simulink model "sourceLocalization_ol"  (R2020a)
settings: Solver=VariableStepAuto  StartTime=0.0  StopTime=inf  RelTol=1e-3
model workspace (MAT data in the model file):
  VADThreshold = 0.5
  c0 = 348
  elementSpace = 0.275
  frameLength = 9600
  fs = 96000
undefined symbols (not defined in the file or in its folder): phased
libraries: dspnetwork x6, audiomeasurements x4, dspstat3 x2, audiosources x1, dspsnks4 x1, dspsrcs4 x1, dspvision x1, dspsigops x1, simulink x1
settings Model: OrderedModelArguments=off  Creator=GH  LastModifiedBy=GH
settings DebuggingCC: UnderSpecifiedDimensionMsg=warning

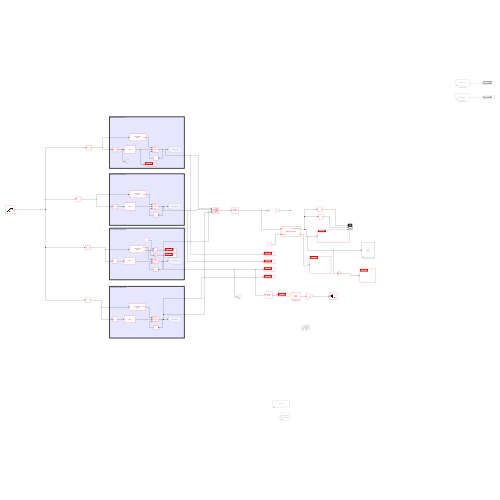
[thumbnail: Simulink's stored preview of the top-level diagram]
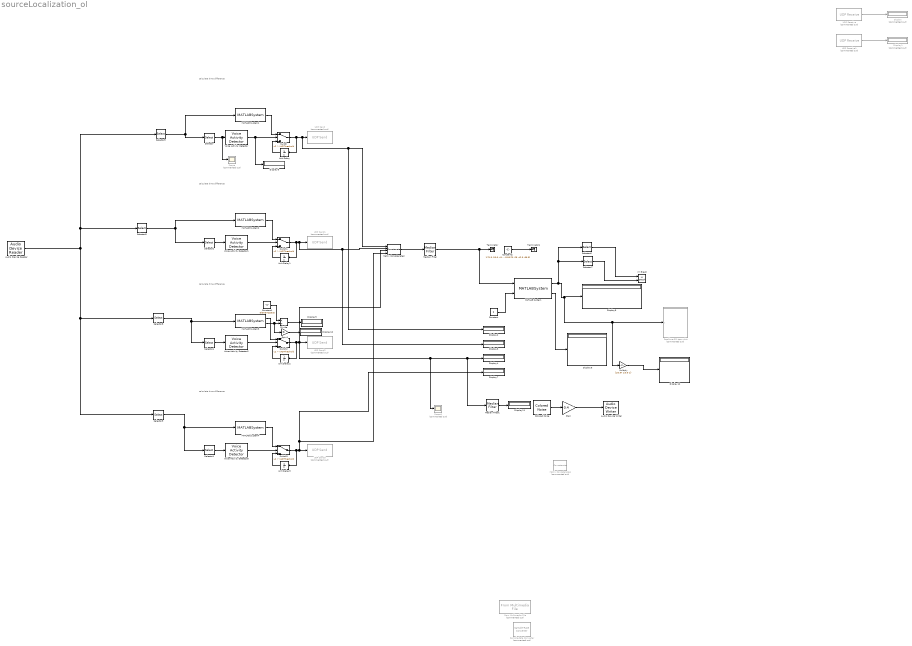
== system sourceLocalization_ol ==
  note: calculate time difference
  note: calculate time difference
  note: calculate time difference
  note: calculate time difference
  Audio Device Reader : audiosources/Audio Device Reader  Driver=ASIO  Device=Default  SampleRate=fs  NumChannels=8  SamplesPerFrame=frameLength  BitDepth=16-bit integer  NumBuffers=10  DefaultInputChannelMapping=on  InputChannelMapping=1:2  OutputNumOverrunSamples=off  OutputDataType=double  DriverIdx=3  DeviceWarnFlag=''
      settings: SourceProductBaseCode=AU
  Audio Device Writer : dspsnks4/Audio Device Writer  Driver=ASIO  Device=Default  InheritSampleRate=on  SampleRate=44100  BitDepth=16-bit integer  BufferSize=4096  NumBuffers=10  DefaultOutputChannelMapping=on  OutputChannelMapping=1:2  OutputNumUnderrunSamples=off  DriverIdx=3  DeviceWarnFlag=''
  Colored Noise : dspsrcs4/Colored Noise  Color=pink  InverseFrequencyPower=1  BoundedOutput=on  NumChannels=1  OutputDataType=double  SamplesPerFrame=frameLength  SampleTime=1/fs  RandomStream=mt19937ar with seed  Seed=67  SimulateUsing=Interpreted execution
      settings: SourceProductBaseCode=DS
  Constant : Constant
  Constant1 : Constant  Value=elementSpace
  Constant2 : Constant  Value=1*[1.5 -26.6 -41.4 -57.9]+0*[0 -28 -42.9 -56.9]  VectorParams1D=off
  Display : Display  Commented=on
  Display1 : Display  Commented=on
  Display{2..12} (11 alike) : Display
  Divide : Product  Inputs=*/
  From Multimedia File : dspvision/From Multimedia File  Commented=on  inputFilename=/Users/developer/Downloads/tan.wav  readRange=[1 Inf]  loop=on  numPlays=inf  outputStreams=Audio only  videoDataType=single  audioDataType=double  inheritSampleTime=on  userDefinedSampleTime=1/30  noAudioOutput=off  isIntensityVideo=off  fourcc=RGB  colorVideoFormat=Separate color signals  outputEOF=off  dataOrg=Column-major  audioFrameSize=frameLength  computeAudioFrameSize=off  outSamplingMode=Sample based
  Gain : Gain  Gain=0.4
  Gain1 : Gain  Gain=fs
  MATLAB System : MATLABSystem  System=getSourcePosition  arrayPos=arrayPos  arrayAxis=arrayAxis  maxStepLength=0.1  sourcePos0=[2;5;2]  SimulateUsing=Interpreted execution
      mask Type: getSourcePosition
      mask Display:
      | disp('getSourcePosition');
      | port_label('input',1,'aoa');
      | port_label('input',2,'calFlag');
      | port_label('output',1,'sourcePosition');
      | port_label('output',2,'dr');
  MATLAB System1 : MATLABSystem  System=GCCEstimator  PropagationSpeed=c0  SampleRateFromInputCheckbox=on  SampleRate=1e6  SensorPairSource=Auto  SensorPair=[ 2; 1 ]  CorrelationOutputPort=off  DelayOutputPort=off  SimulateUsing=Interpreted execution  SensorArray=phased.ULA('Element',phased.OmnidirectionalMicrophoneElement(),'ElementSpacing',elementSpace)
      mask Type: GCCEstimator
      mask Display:
      | disp(['GCC-PHAT' char(10) 'DOA']);
      | port_label('output',1,'Ang');
  MATLAB System2 : MATLABSystem  System=GCCEstimator  PropagationSpeed=c0  SampleRateFromInputCheckbox=on  SampleRate=1e6  SensorPairSource=Auto  SensorPair=[ 2; 1 ]  CorrelationOutputPort=off  DelayOutputPort=off  SimulateUsing=Interpreted execution  SensorArray=phased.ULA('Element',phased.OmnidirectionalMicrophoneElement(),'ElementSpacing',elementSpace)
      mask Type: GCCEstimator
      mask Display:
      | disp(['GCC-PHAT' char(10) 'DOA']);
      | port_label('output',1,'Ang');
  MATLAB System3 : MATLABSystem  System=GCCEstimator  PropagationSpeed=c0  SampleRateFromInputCheckbox=on  SampleRate=1e6  SensorPairSource=Auto  SensorPair=[ 2; 1 ]  CorrelationOutputPort=off  DelayOutputPort=on  SimulateUsing=Interpreted execution  SensorArray=phased.ULA('Element',phased.OmnidirectionalMicrophoneElement(),'ElementSpacing',elementSpace)
      mask Type: GCCEstimator
      mask Display:
      | disp(['GCC-PHAT' char(10) 'DOA']);
      | port_label('output',1,'Ang');
      | port_label('output',2,'Tau');
  MATLAB System4 : MATLABSystem  System=GCCEstimator  PropagationSpeed=c0  SampleRateFromInputCheckbox=on  SampleRate=1e6  SensorPairSource=Auto  SensorPair=[ 2; 1 ]  CorrelationOutputPort=off  DelayOutputPort=off  SimulateUsing=Interpreted execution  SensorArray=phased.ULA('Element',phased.OmnidirectionalMicrophoneElement(),'ElementSpacing',elementSpace)
      mask Type: GCCEstimator
      mask Display:
      | disp(['GCC-PHAT' char(10) 'DOA']);
      | port_label('output',1,'Ang');
  Matrix Concatenate1 : Concatenate  Commented=on  Mode=Multidimensional array  ConcatenateDimension=2
  Matrix Concatenate2 : Concatenate  NumInputs=4  Mode=Multidimensional array  ConcatenateDimension=2
  Median Filter : dspstat3/Median Filter  WindowLength=3  SimulateUsing=Interpreted execution
      settings: SourceProductBaseCode=DS
  Median Filter1 : dspstat3/Median Filter  WindowLength=3  SimulateUsing=Interpreted execution
      settings: SourceProductBaseCode=DS
  Multiply : Gain  Gain=[1/0.97 1/0.9 1]'
  Realtime-3D stem plot : MATLAB Function  Commented=on  TreatAsAtomicUnit=on
  Sample-Rate Converter : dspsigops/Sample-Rate Converter  Commented=on  InputSampleRate=48e3  OutputSampleRate=fs  OutputRateTolerance=0  Bandwidth=40e3  StopbandAttenuation=80  SimulateUsing=Code generation
      settings: SourceProductBaseCode=DS
  Scope : Scope  Commented=on
  Scope1 : Scope  Commented=on
  Selector{,1..2,4} (4 alike) : Selector  NumberOfDimensions=2  InputPortWidth=3  IndexOptions=Select all,Index vector (dialog)  Indices=[1 3],1  OutputSizes=1,1
  Selector3 : Selector  NumberOfDimensions=2  InputPortWidth=3  IndexOptions=Select all,Index vector (dialog)  Indices=[1 3],[1 2]  OutputSizes=1,1
  Selector5 : Selector  NumberOfDimensions=2  InputPortWidth=3  IndexOptions=Select all,Index vector (dialog)  Indices=[1 3],[3 4]  OutputSizes=1,1
  Selector6 : Selector  NumberOfDimensions=2  InputPortWidth=3  IndexOptions=Index vector (dialog),Select all  Indices=1,[1 2]  OutputSizes=1,1
  Selector7 : Selector  NumberOfDimensions=2  InputPortWidth=3  IndexOptions=Index vector (dialog),Select all  Indices=2,[1 2]  OutputSizes=1,1
  Selector8 : Selector  NumberOfDimensions=2  InputPortWidth=3  IndexOptions=Select all,Index vector (dialog)  Indices=[1 3],[5 6]  OutputSizes=1,1
  Selector9 : Selector  NumberOfDimensions=2  InputPortWidth=3  IndexOptions=Select all,Index vector (dialog)  Indices=[1 3],[7 8]  OutputSizes=1,1
  Switch{,1..3} (4 alike) : Switch  Criteria=u2 > Threshold  Threshold=VADThreshold
  Terminator : Terminator
  Terminator1 : Terminator
  UDP Receive : dspnetwork/UDP Receive  Commented=on  localURL='0.0.0.0'  localPort=23450  remoteURL='0.0.0.0'  remotePort=-1  recvBufferSize=8192  dims=255  signalDatatype=double  isComplex=off  isVarSize=on  showBlockingTime=off  blockingTime=0  sampletime=frameLength/fs  blockPlatform=[]
  UDP Receive1 : dspnetwork/UDP Receive  Commented=on  localURL='0.0.0.0'  localPort=23451  remoteURL='0.0.0.0'  remotePort=-1  recvBufferSize=8192  dims=255  signalDatatype=double  isComplex=off  isVarSize=on  showBlockingTime=off  blockingTime=0  sampletime=frameLength/fs  blockPlatform=[]
  UDP Send : dspnetwork/UDP Send  Commented=on  remoteURL='127.0.0.1'  remotePort=23450  localURL='0.0.0.0'  localPortSource=Automatically determine  localPort=-1  sendBufferSize=8192  sampletime=-1  blockPlatform=[]  separateLengthPort=0
  UDP Send1 : dspnetwork/UDP Send  Commented=on  remoteURL='127.0.0.1'  remotePort=23451  localURL='0.0.0.0'  localPortSource=Automatically determine  localPort=-1  sendBufferSize=8192  sampletime=-1  blockPlatform=[]  separateLengthPort=0
  UDP Send2 : dspnetwork/UDP Send  Commented=on  remoteURL='127.0.0.1'  remotePort=23452  localURL='0.0.0.0'  localPortSource=Automatically determine  localPort=-1  sendBufferSize=8192  sampletime=-1  blockPlatform=[]  separateLengthPort=0
  UDP Send3 : dspnetwork/UDP Send  Commented=on  remoteURL='127.0.0.1'  remotePort=23452  localURL='0.0.0.0'  localPortSource=Automatically determine  localPort=-1  sendBufferSize=8192  sampletime=-1  blockPlatform=[]  separateLengthPort=0
  Unit Delay{,1..3} (4 alike) : UnitDelay  InputProcessing=Columns as channels (frame based)  SampleTime=-1  HasFrameUpgradeWarning=on
  Voice Activity Detector{,1..3} (4 alike) : audiomeasurements/Voice Activity Detector  InputDomain=Time  Window=Hann  SidelobeAttenuation=60  InheritFFTLength=on  FFTLength=1024  SilenceToSpeechProbabilityPort=off  SilenceToSpeechProbability=0.2  SpeechToSilenceProbabilityPort=off  SpeechToSilenceProbability=0.1  OutputNoiseVariance=off  SimulateUsing=Code generation
      settings: SourceProductBaseCode=AU
  XY Graph : simulink/Sinks/XY Graph  xmin=-1  xmax=1  ymin=-1  ymax=1  st=-1
  wires:
  MATLAB System1/1 -> Switch/1
  Voice Activity Detector/1 -> Display8/1, Switch/2
  Switch/1 -> Matrix Concatenate2/1, Display2/1, UDP Send/1, Unit Delay/1
  Unit Delay/1 -> Switch/3
  Selector/1 -> Scope/1, Voice Activity Detector/1
  UDP Receive/1 -> Display/1
  Selector2/1 -> Voice Activity Detector1/1
  Voice Activity Detector1/1 -> Switch1/2
  Unit Delay1/1 -> Switch1/3
  Switch1/1 -> UDP Send1/1, Display3/1, Matrix Concatenate2/2, Unit Delay1/1
  MATLAB System2/1 -> Switch1/1
  UDP Receive1/1 -> Display1/1
  Voice Activity Detector2/1 -> Switch2/2
  Unit Delay2/1 -> Switch2/3
  MATLAB System3/1 -> Switch2/1
  Selector4/1 -> Voice Activity Detector2/1
  Constant/1 -> MATLAB System/2
  MATLAB System/2 -> Display6/1
  Selector6/1 -> XY Graph/1
  Selector7/1 -> XY Graph/2
  Unit Delay3/1 -> Switch3/3
  Selector1/1 -> Voice Activity Detector3/1
  Switch3/1 -> Matrix Concatenate2/4, Display7/1, UDP Send3/1, Unit Delay3/1
  MATLAB System4/1 -> Switch3/1
  Voice Activity Detector3/1 -> Switch3/2
  Audio Device Reader/1 -> Selector9/1, Selector8/1, Selector5/1, Selector3/1
  Selector3/1 -> MATLAB System1/1, Selector/1
  Selector9/1 -> MATLAB System4/1, Selector1/1
  Selector8/1 -> MATLAB System3/1, Selector4/1
  Selector5/1 -> MATLAB System2/1, Selector2/1
  MATLAB System3/2 -> Gain1/1, Divide/2
  Divide/1 -> Display9/1
  Constant1/1 -> Divide/1
  Gain1/1 -> Display10/1
  Colored Noise/1 -> Gain/1
  Constant2/1 -> Terminator1/1
  Gain/1 -> Audio Device Writer/1
  Matrix Concatenate2/1 -> Median Filter/1
  Switch2/1 -> Scope1/1, Median Filter1/1, Display4/1, Matrix Concatenate2/3, UDP Send2/1, Unit Delay2/1
  Median Filter1/1 -> Display11/1
  Multiply/1 -> Display12/1
  MATLAB System/1 -> Selector7/1, Selector6/1, Display5/1, Multiply/1, Realtime-3D stem plot/1(x)
  Median Filter/1 -> MATLAB System/1, Terminator/1

== matlab function sourceLocalization_ol/Realtime-3D stem plot ==
  data: x input
function  fcn(x)
figure(1);
% hold on;
grid on;
coder.extrinsic('stem3');
stem3(1/0.97*x(1), 1/0.9*x(2), x(3));
xlim([0 5]);xlabel(sprintf('x: %f', 1/0.97*x(1)));
ylim([0 6]);ylabel(sprintf('y: %f', 1/0.9*x(2)));
zlim([0 2]);zlabel(sprintf('z: %f', x(3)));
view([45 45]);
